simulink model "ModeloSWa2"  (R2018b)
settings: Solver=VariableStepAuto  StartTime=0.0  StopTime=50  MaxStep=1e-3  RelTol=1e-3
undefined symbols (not defined in the file or in its folder): Tt
libraries: simulink x2
settings Model: Creator=15.01580-7  LastModifiedBy=18.01353-8

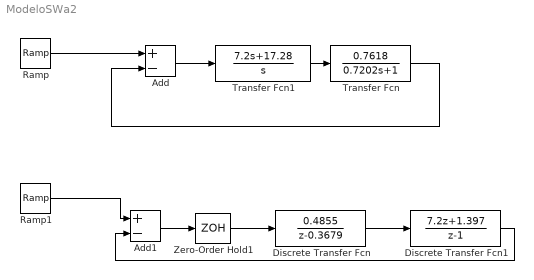
== system ModeloSWa2 ==
  Add : Sum  Inputs=+-
  Add1 : Sum  Inputs=+-
  Discrete Transfer Fcn : DiscreteTransferFcn  Numerator=0.4855  Denominator=[1 -0.3679]  SampleTime=Tt
  Discrete Transfer Fcn1 : DiscreteTransferFcn  Numerator=[7.2 1.397]  Denominator=[1 -1]  SampleTime=Tt
  Ramp : simulink/Sources/Ramp  slope=1  start=0  InitialOutput=0
  Ramp1 : simulink/Sources/Ramp  slope=1  start=0  InitialOutput=0
  Transfer Fcn : TransferFcn  Numerator=0.7618  Denominator=[0.7202 1]
  Transfer Fcn1 : TransferFcn  Numerator=[7.2 17.28]  Denominator=[1 0]
  Zero-Order Hold1 : ZeroOrderHold  SampleTime=Tt
  wires:
  Ramp/1 -> Add/1
  Transfer Fcn/1 -> Add/2
  Add/1 -> Transfer Fcn1/1
  Transfer Fcn1/1 -> Transfer Fcn/1
  Discrete Transfer Fcn1/1 -> Add1/2
  Add1/1 -> Zero-Order Hold1/1
  Discrete Transfer Fcn/1 -> Discrete Transfer Fcn1/1
  Ramp1/1 -> Add1/1
  Zero-Order Hold1/1 -> Discrete Transfer Fcn/1
